simulink model "Sim5"  (R2021b)
settings: Solver=VariableStepAuto  StartTime=0.0  StopTime=1.0  RelTol=1e-3
libraries: slpidlib x1, spsPLL3phLib x1, spsabctodq0Lib x1
settings Model: Creator=sebastian  LastModifiedBy=sebastian

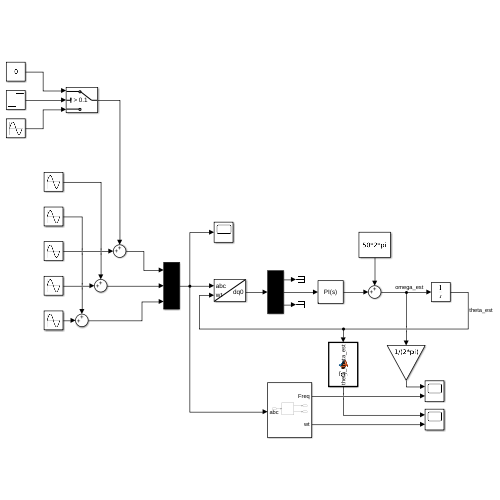
[thumbnail: Simulink's stored preview of the top-level diagram]
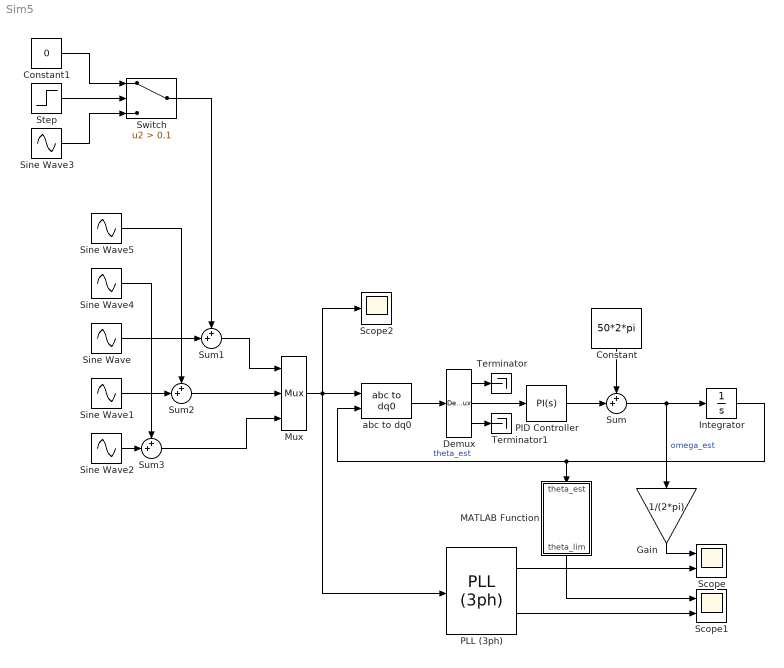
== system Sim5 ==
  Constant : Constant  Value=50*2*pi
  Constant1 : Constant  Value=0
  Demux : Demux  Outputs=3
  Gain : Gain  Gain=1/(2*pi)
  Integrator : Integrator
  MATLAB Function : MATLAB Function  TreatAsAtomicUnit=on
  Mux : Mux  Inputs=3
  PID Controller : slpidlib/PID Controller  Controller=PI  Form=Parallel  TimeDomain=Continuous-time  UseExternalTs=off  SampleTime=-1  IntegratorMethod=Forward Euler  FilterMethod=Forward Euler  ControllerParametersSource=internal  P=0.001  I=0.001  D=0  UseFilter=on  N=100  TunerSelectOption=Transfer Function Based (PID Tuner App)  InitialConditionSource=internal  InitialConditionForIntegrator=0  InitialConditionForFilter=0  DifferentiatorICPrevScaledInput=0  ExternalReset=none  TrackingMode=off  Kt=1  LimitOutput=off  SatLimitsSource=internal  UpperSaturationLimit=inf  LowerSaturationLimit=-inf  LinearizeAsGain=on  AntiWindupMode=none  Kb=1  POutMin=[]  POutMax=[]  IOutMin=[]  IOutMax=[]  DOutMin=[]  DOutMax=[]  NOutMin=[]  NOutMax=[]  SumOutMin=[]  SumOutMax=[]  SaturationOutMin=[]  SaturationOutMax=[]  PParamMin=[]  PParamMax=[]  IParamMin=[]  IParamMax=[]  DParamMin=[]  DParamMax=[]  NParamMin=[]  NParamMax=[]  KbParamMin=[]  KbParamMax=[]  KtParamMin=[]  KtParamMax=[]  KbOutMin=[]  KbOutMax=[]  KtOutMin=[]  KtOutMax=[]  IntegratorOutMin=[]  IntegratorOutMax=[]  FilterOutMin=[]  FilterOutMax=[]  SumI1OutMin=[]  SumI1OutMax=[]  SumI2OutMin=[]  SumI2OutMax=[]  SumI3OutMin=[]  SumI3OutMax=[]  SumI4OutMin=[]  SumI4OutMax=[]  SumDOutMin=[]  SumDOutMax=[]  DifferentiatorOutMin=[]  DifferentiatorOutMax=[]  FilterDiffOutCoefMin=[]  FilterDiffOutCoefMax=[]  ReciprocalOutMin=[]  ReciprocalOutMax=[]  SumDenOutMin=[]  SumDenOutMax=[]  SumNumOutMin=[]  SumNumOutMax=[]  DivideOutMin=[]  DivideOutMax=[]  UdiffTsProdOutMin=[]  UdiffTsProdOutMax=[]  NTsProdOutMin=[]  NTsProdOutMax=[]  UintegralTsProdOutMin=[]  UintegralTsProdOutMax=[]  UngainTsProdOutMin=[]  UngainTsProdOutMax=[]  IntegratorContinuousStateAttributes=''  IntegratorStateMustResolveToSignalObject=off  IntegratorRTWStateStorageClass=Auto  FilterContinuousStateAttributes=''  FilterStateMustResolveToSignalObject=off  FilterRTWStateStorageClass=Auto  ParallelPVariant=InternalParameters  IdealPVariant=Disabled  IVariant=InternalParameters  DVariant=Disabled  IntegratorVariant=Continuous  SatVariant=Disabled  AWVariant=Passthrough  PCopyVariant=Disabled  TRVariant=Disabled  FdbkBlocksVariant=Forward  IdealPFdbkVariant=Disabled  SatFdbkVariant=Disabled  DerivativeFilterVariant=Disabled  NVariant=Disabled  NCopyVariant=Disabled_SignalSpec  FilterICVariant=Disabled  IntegratorICVariant=InternalICs  ExternalResetVariant=Disabled  TRSumVariant=Passthrough  SumFdbkVariant=Disabled  SumVariant=Sum_PI  TsampFilterVariant=InternalTs  TsampNgainVariant=Passthrough  TsampIntegralVariant=Passthrough  ExternalSaturationOutDataTypeStr=Inherit: Same as second input
  PLL (3ph) : spsPLL3phLib/PLL (3ph)  Fmin=45  Par_Init=[0, 50]  ParK=[180, 3200, 1]  TcD=1e-4  MaxRateChangeFreq=12  FilterCutOffFreq=25  Ts=0  AGC=on
  Scope : Scope  NumInputPorts=2
  Scope1 : Scope  NumInputPorts=2
  Scope2 : Scope
  Sine Wave : Sin  Amplitude=230  Frequency=50*2*pi  SampleTime=0
  Sine Wave1 : Sin  Amplitude=230  Frequency=50*2*pi  Phase=-2*pi/3  SampleTime=0
  Sine Wave2 : Sin  Amplitude=230  Frequency=50*2*pi  Phase=2*pi/3  SampleTime=0
  Sine Wave3 : Sin  Amplitude=15  Frequency=250*2*pi  SampleTime=0
  Sine Wave4 : Sin  Amplitude=20  Frequency=450*2*pi  SampleTime=0
  Sine Wave5 : Sin  Amplitude=20  Frequency=350*2*pi  SampleTime=0
  Step : Step  Time=0.1  SampleTime=0
  Sum{,1..3} (4 alike) : Sum  Inputs=++|
  Switch : Switch  Criteria=u2 > Threshold  Threshold=0.1
  Terminator : Terminator
  Terminator1 : Terminator
  abc to dq0 : spsabctodq0Lib/abc to dq0  Alignment=90 degrees behind phase A axis
  wires:
  Mux/1 -> Scope2/1, PLL (3ph)/1, abc to dq0/1
  PID Controller/1 -> Sum/2
  Constant/1 -> Sum/1
  Sum/1 -> Integrator/1, Gain/1  "omega_est"
  Integrator/1 -> MATLAB Function/1(theta_est), abc to dq0/2  "theta_est"
  PLL (3ph)/1 -> Scope/2
  PLL (3ph)/2 -> Scope1/2
  abc to dq0/1 -> Demux/1
  Demux/2 -> PID Controller/1
  Demux/1 -> Terminator/1
  Demux/3 -> Terminator1/1
  Gain/1 -> Scope/1
  MATLAB Function/1(theta_lim) -> Scope1/1
  Sine Wave/1 -> Sum1/2
  Sum1/1 -> Mux/1
  Sine Wave2/1 -> Sum3/2
  Sine Wave1/1 -> Sum2/2
  Sum2/1 -> Mux/2
  Sum3/1 -> Mux/3
  Sine Wave5/1 -> Sum2/1
  Sine Wave4/1 -> Sum3/1
  Sine Wave3/1 -> Switch/3
  Switch/1 -> Sum1/1
  Constant1/1 -> Switch/1
  Step/1 -> Switch/2

== matlab function Sim5/MATLAB Function ==
  data: theta_est input; theta_lim output
function theta_lim = fcn(theta_est)

theta_lim = theta_est;

while theta_lim >= 2*pi
    theta_lim = theta_lim - 2*pi;
end
while theta_lim < 0
    theta_lim = theta_lim + 2*pi;
end
